simulink model "interpolated"  (R2022a)
settings: Solver=VariableStepAuto  StartTime=0.0  StopTime=5  RelTol=1e-3
undefined symbols (not defined in the file or in its folder): k_int, K_int_matrix
settings Model: Creator=mihai  LastModifiedBy=mihai

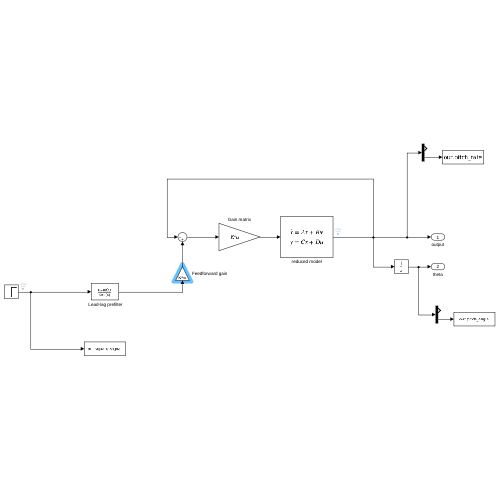
[thumbnail: Simulink's stored preview of the top-level diagram]
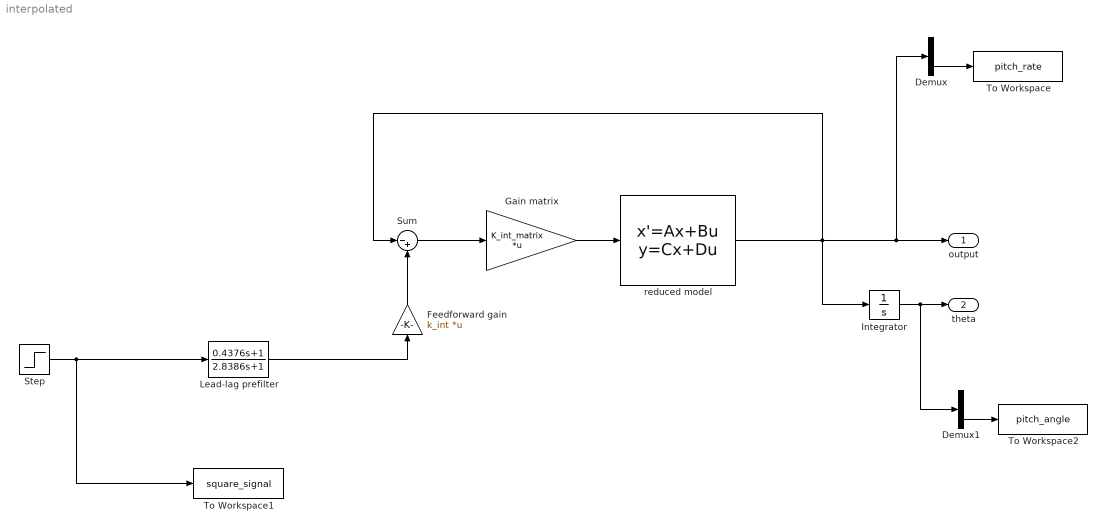
== system interpolated ==
  " Lead-lag prefilter" : TransferFcn  Numerator=[0.4376, 1]  Denominator=[2.8386, 1]
  Demux : Demux  Outputs=2
  Demux1 : Demux  Outputs=2
  Feedforward gain : Gain  Gain=k_int  Multiplication=Matrix(K*u)
  Gain matrix : Gain  Gain=K_int_matrix  Multiplication=Matrix(K*u)
  Integrator : Integrator
  Step : Step  Time=0  OutDataTypeStr=Inherit: Inherit via back propagation  SampleTime=0
  Sum : Sum  Inputs=|-+
  To Workspace : ToWorkspace  VariableName=pitch_rate  SaveFormat=Timeseries  SampleTime=-1
  To Workspace1 : ToWorkspace  VariableName=square_signal  SaveFormat=Timeseries  SampleTime=-1
  To Workspace2 : ToWorkspace  VariableName=pitch_angle  SaveFormat=Timeseries  SampleTime=-1
  reduced model : StateSpace  A=[-0.3821, 0.9481; 0.2462, -0.5939]  B=[-0.0008; -0.0484]  C=[57.2958, 0; 0, 57.2958]  D=[0; 0]  InitialCondition=0
  output : Outport
  theta : Outport  Port=2
  wires:
  Gain matrix/1 -> reduced model/1
  Sum/1 -> Gain matrix/1
  Step/1 -> To Workspace1/1, " Lead-lag prefilter"/1
  " Lead-lag prefilter"/1 -> Feedforward gain/1
  Feedforward gain/1 -> Sum/2
  Integrator/1 -> theta/1, Demux1/1
  reduced model/1 -> Demux/1, output/1, Integrator/1, Sum/1
  Demux1/2 -> To Workspace2/1
  Demux/2 -> To Workspace/1
